simulink model "summary"  (R2022b)
settings: Solver=FixedStepAuto  StartTime=0.0  StopTime=100  FixedStep=0.1  RelTol=1e-3
values from neighbouring files (symbols this model uses):
  C_M = 1.1366    [init.m]
  C_T = 3.5611    [init.m]
  D_p = 0.1    [init.m]
  ModelInit_Att_qw = 0    [init.m]
  ModelInit_Att_qx = 1    [init.m]
  ModelInit_Att_qy = 0    [init.m]
  ModelInit_Att_qz = 0    [init.m]
  ModelInit_Pos_x = 0    [init.m]
  ModelInit_Pos_y = 0    [init.m]
  ModelInit_Pos_z = 0    [init.m]
  ModelParam_c_M = 1.779e-07*2    (= 3.558e-07)    [init.m]
  ModelParam_c_T = 1.105e-05    [init.m]
  ModelParam_d = 0.225    [init.m]
  ModelParam_g = 9.8    [init.m]
  ModelParam_I_xx = 0.0211    [init.m]
  ModelParam_I_yy = 0.0219    [init.m]
  ModelParam_I_zz = 0.0366    [init.m]
  ModelParam_J_RP = 0.0001287    [init.m]
  ModelParam_m = 1.4    [init.m]
  p = pos(idx,:)    [draw_morecool.m]    (also in init.m = 1.225)
libraries: mpclib x3
settings Model: Creator=12854  LastModifiedBy=12854
settings OptimizationCC: BlockReduction=off  DefaultParameterBehavior=Inlined  BufferReuse=off

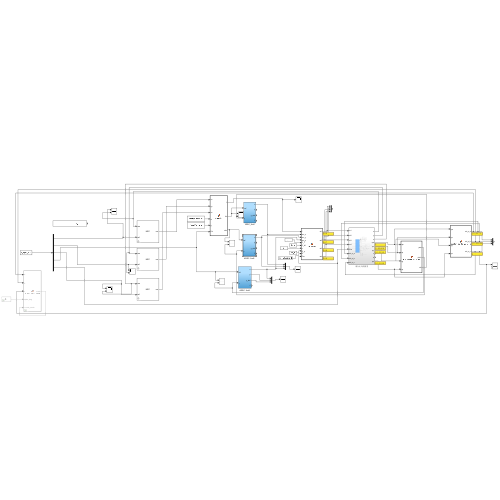
[thumbnail: Simulink's stored preview of the top-level diagram]
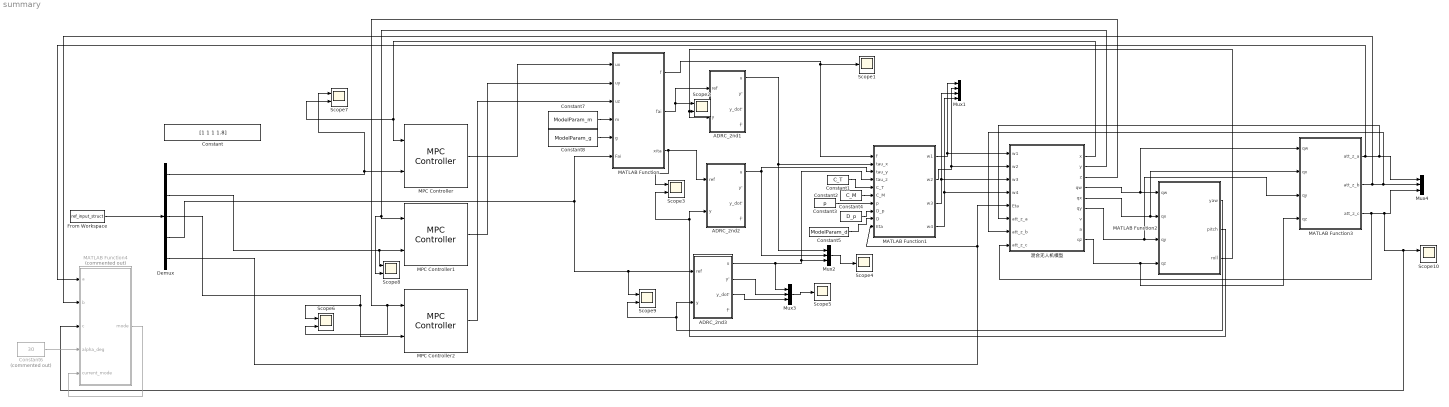
== system summary ==
  ADRC_2nd1 : Subsystem
  ADRC_2nd2 : Subsystem
  ADRC_2nd3 : Subsystem
  Constant : Constant  Value=[1 1 1 1.8]
  Constant1 : Constant  Value=C_T
  Constant2 : Constant  Value=C_M
  Constant3 : Constant  Value=p
  Constant4 : Constant  Value=D_p
  Constant5 : Constant  Value=ModelParam_d
  Constant6 : Constant  Commented=on  Value=30
  Constant7 : Constant  Value=ModelParam_m
  Constant8 : Constant  Value=ModelParam_g
  Demux : Demux  Outputs=5
  From Workspace : FromWorkspace  VariableName=ref_input_struct
  MATLAB Function : MATLAB Function  TreatAsAtomicUnit=on
  MATLAB Function1 : MATLAB Function  TreatAsAtomicUnit=on
  MATLAB Function2 : MATLAB Function  TreatAsAtomicUnit=on
  MATLAB Function3 : MATLAB Function  TreatAsAtomicUnit=on
  MATLAB Function4 : MATLAB Function  Commented=on  TreatAsAtomicUnit=on
  MPC Controller : mpclib/MPC Controller  SCDEnableBlockLinearizationSpecification=on  mpcobj=mpcobj_x  x0=[]  is_multiple=0  enable_value=0  return_u0=off  updateMPCinCallerWorkspace=on  md_inport=off  mv_inport=off  uref_inport=off  return_cost=off  return_mvseq=off  return_qpstatus=off  return_xseq=off  return_state=off  return_ovseq=off  state_inport=off  umin_inport=off  umax_inport=off  ymin_inport=off  ymax_inport=off  cc_inport=off  ywt_inport=off  uwt_inport=off  duwt_inport=off  rhoeps_inport=off  pm_inport=off  MaximumP=10  HorizonChoice=FixedHorizon  n_ts=0.1  n_p=10  n_mv=1  n_md=0  n_ud=0  n_mo=1  n_uo=0  BlockDataType=double  SampleTimeInherited=off  switch_inport=off
  MPC Controller1 : mpclib/MPC Controller  SCDEnableBlockLinearizationSpecification=on  mpcobj=mpcobj_y  x0=[]  is_multiple=0  enable_value=0  return_u0=off  updateMPCinCallerWorkspace=on  md_inport=off  mv_inport=off  uref_inport=off  return_cost=off  return_mvseq=off  return_qpstatus=off  return_xseq=off  return_state=off  return_ovseq=off  state_inport=off  umin_inport=off  umax_inport=off  ymin_inport=off  ymax_inport=off  cc_inport=off  ywt_inport=off  uwt_inport=off  duwt_inport=off  rhoeps_inport=off  pm_inport=off  MaximumP=10  HorizonChoice=FixedHorizon  n_ts=0.1  n_p=10  n_mv=1  n_md=0  n_ud=0  n_mo=1  n_uo=0  BlockDataType=double  SampleTimeInherited=off  switch_inport=off
  MPC Controller2 : mpclib/MPC Controller  SCDEnableBlockLinearizationSpecification=on  mpcobj=mpcobj_z  x0=[]  is_multiple=0  enable_value=0  return_u0=off  updateMPCinCallerWorkspace=on  md_inport=off  mv_inport=off  uref_inport=off  return_cost=off  return_mvseq=off  return_qpstatus=off  return_xseq=off  return_state=off  return_ovseq=off  state_inport=off  umin_inport=off  umax_inport=off  ymin_inport=off  ymax_inport=off  cc_inport=off  ywt_inport=off  uwt_inport=off  duwt_inport=off  rhoeps_inport=off  pm_inport=off  MaximumP=10  HorizonChoice=FixedHorizon  n_ts=0.1  n_p=10  n_mv=1  n_md=0  n_ud=0  n_mo=1  n_uo=0  BlockDataType=double  SampleTimeInherited=off  switch_inport=off
  Mux1 : Mux
  Mux2 : Mux  Inputs=3
  Mux3 : Mux  Inputs=3
  Mux4 : Mux  Inputs=3
  Scope1 : Scope
  Scope{2..3,6..10} (7 alike) : Scope  NumInputPorts=2
  Scope4 : Scope
  Scope5 : Scope
  混合无人机模型 : Subsystem
  wires:
  混合无人机模型/1(x) -> MPC Controller/1, Scope7/2
  混合无人机模型/2(y) -> Scope8/2, MPC Controller1/1
  混合无人机模型/3(z) -> Scope6/2, MPC Controller2/1
  Demux/1 -> Scope7/1, MPC Controller/2
  Demux/2 -> Scope8/1, MPC Controller1/2
  Demux/3 -> Scope6/1, MPC Controller2/2
  From Workspace/1 -> Demux/1
  MPC Controller/1 -> MATLAB Function/1(ux)
  MPC Controller1/1 -> MATLAB Function/2(uy)
  MPC Controller2/1 -> MATLAB Function/3(uz)
  Demux/4 -> MATLAB Function/6(Fai), Scope9/1, ADRC_2nd3/1(ref)
  Constant8/1 -> MATLAB Function/5(g)
  Constant7/1 -> MATLAB Function/4(m)
  MATLAB Function/1(f) -> Scope1/1, MATLAB Function1/1(f)
  MATLAB Function/2(fai) -> ADRC_2nd1/1(ref), Scope2/1
  MATLAB Function/3(xita) -> ADRC_2nd2/1(ref), Scope3/1
  ADRC_2nd3/1(u) -> Mux2/3, MATLAB Function1/4(tau_z), Mux3/1
  MATLAB Function1/1(w1) -> Mux1/1, 混合无人机模型/1(w1)
  MATLAB Function1/2(w2) -> 混合无人机模型/2(w2), Mux1/2
  MATLAB Function1/3(w3) -> 混合无人机模型/3(w3), Mux1/3
  MATLAB Function1/4(w4) -> 混合无人机模型/4(w4), Mux1/4
  Constant1/1 -> MATLAB Function1/5(C_T)
  Constant2/1 -> MATLAB Function1/6(C_M)
  Constant4/1 -> MATLAB Function1/8(D_p)
  Constant5/1 -> MATLAB Function1/9(D)
  Mux2/1 -> Scope4/1
  Mux3/1 -> Scope5/1
  ADRC_2nd3/2(y') -> Mux3/2
  ADRC_2nd3/3(y_dot') -> Mux3/3
  ADRC_2nd1/1(u) -> Mux2/1, MATLAB Function1/2(tau_x)
  ADRC_2nd2/1(u) -> Mux2/2, MATLAB Function1/3(tau_y)
  Constant3/1 -> MATLAB Function1/7(p)
  Demux/5 -> MATLAB Function1/10(Eta), 混合无人机模型/5(Eta)
  混合无人机模型/4(qw) -> MATLAB Function3/1(qw), MATLAB Function2/1(qw)
  混合无人机模型/5(qx) -> MATLAB Function3/2(qx), MATLAB Function2/2(qx)
  混合无人机模型/6(qy) -> MATLAB Function3/3(qy), MATLAB Function2/3(qy)
  混合无人机模型/9(qz) -> MATLAB Function3/4(qz), MATLAB Function2/4(qz)
  MATLAB Function2/3(roll) -> Scope2/2, ADRC_2nd1/2(y)
  MATLAB Function2/2(pitch) -> Scope3/2, ADRC_2nd2/2(y)
  MATLAB Function2/1(yaw) -> Scope9/2, ADRC_2nd3/2(y)
  MATLAB Function3/2(att_z_b) -> MATLAB Function4/2(b), 混合无人机模型/7(att_z_b), Mux4/2
  MATLAB Function3/3(att_z_c) -> 混合无人机模型/8(att_z_c), MATLAB Function4/3(c), Scope10/1, Mux4/3
  MATLAB Function4/1(mode) -> MATLAB Function4/5(current_mode)
  MATLAB Function3/1(att_z_a) -> MATLAB Function4/1(a), 混合无人机模型/6(att_z_a), Mux4/1
  Constant6/1 -> MATLAB Function4/4(alpha_deg)

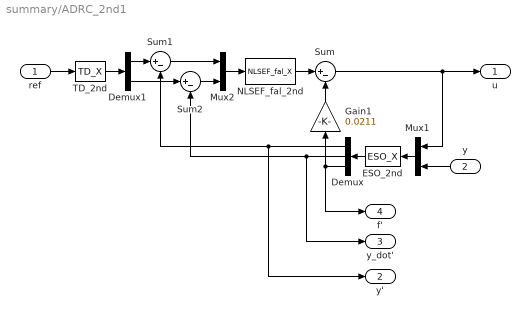
== system summary/ADRC_2nd1 ==
  ref : Inport
  y : Inport  Port=2
  Demux : Demux  Outputs=3
  Demux1 : Demux  Outputs=2
  ESO_2nd : S-Function  FunctionName=ESO_X  Parameters=CtrlParaX  SFunctionDeploymentMode=off  EnableBusSupport=off
  Gain1 : Gain  Gain=0.0211
  Mux1 : Mux  Inputs=2
  Mux2 : Mux  Inputs=2
  NLSEF_fal_2nd : S-Function  FunctionName=NLSEF_fal_X  Parameters=CtrlParaX  SFunctionDeploymentMode=off  EnableBusSupport=off
  Sum : Sum  Inputs=|+-
  Sum1 : Sum  Inputs=|+-
  Sum2 : Sum  Inputs=|+-
  TD_2nd : S-Function  FunctionName=TD_X  Parameters=CtrlParaX  SFunctionDeploymentMode=off  EnableBusSupport=off
  u : Outport  VectorParamsAs1DForOutWhenUnconnected=off
  y' : Outport  Port=2  VectorParamsAs1DForOutWhenUnconnected=off
  y_dot' : Outport  Port=3  VectorParamsAs1DForOutWhenUnconnected=off
  f' : Outport  Port=4  VectorParamsAs1DForOutWhenUnconnected=off
  wires:
  Mux2/1 -> NLSEF_fal_2nd/1
  ESO_2nd/1 -> Demux/1
  Demux1/2 -> Sum2/1
  ref/1 -> TD_2nd/1
  Demux/1 -> y'/1, Sum1/2
  TD_2nd/1 -> Demux1/1
  y/1 -> Mux1/2
  Gain1/1 -> Sum/2
  Demux/2 -> y_dot'/1, Sum2/2
  Demux1/1 -> Sum1/1
  Demux/3 -> Gain1/1, f'/1
  Sum2/1 -> Mux2/2
  Sum/1 -> Mux1/1, u/1
  NLSEF_fal_2nd/1 -> Sum/1
  Sum1/1 -> Mux2/1
  Mux1/1 -> ESO_2nd/1

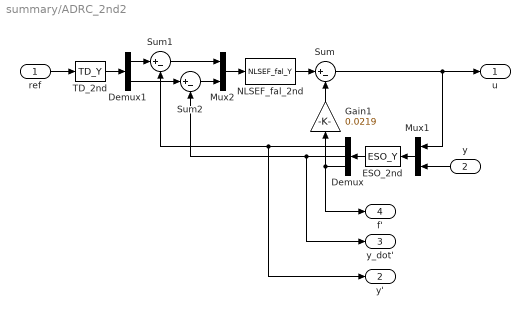
== system summary/ADRC_2nd2 ==
  ref : Inport
  y : Inport  Port=2
  Demux : Demux  Outputs=3
  Demux1 : Demux  Outputs=2
  ESO_2nd : S-Function  FunctionName=ESO_Y  Parameters=CtrlParaY  SFunctionDeploymentMode=off  EnableBusSupport=off
  Gain1 : Gain  Gain=0.0219
  Mux1 : Mux  Inputs=2
  Mux2 : Mux  Inputs=2
  NLSEF_fal_2nd : S-Function  FunctionName=NLSEF_fal_Y  Parameters=CtrlParaY  SFunctionDeploymentMode=off  EnableBusSupport=off
  Sum : Sum  Inputs=|+-
  Sum1 : Sum  Inputs=|+-
  Sum2 : Sum  Inputs=|+-
  TD_2nd : S-Function  FunctionName=TD_Y  Parameters=CtrlParaY  SFunctionDeploymentMode=off  EnableBusSupport=off
  u : Outport  VectorParamsAs1DForOutWhenUnconnected=off
  y' : Outport  Port=2  VectorParamsAs1DForOutWhenUnconnected=off
  y_dot' : Outport  Port=3  VectorParamsAs1DForOutWhenUnconnected=off
  f' : Outport  Port=4  VectorParamsAs1DForOutWhenUnconnected=off
  wires:
  Mux2/1 -> NLSEF_fal_2nd/1
  ESO_2nd/1 -> Demux/1
  Demux1/2 -> Sum2/1
  ref/1 -> TD_2nd/1
  Demux/1 -> y'/1, Sum1/2
  TD_2nd/1 -> Demux1/1
  y/1 -> Mux1/2
  Gain1/1 -> Sum/2
  Demux/2 -> y_dot'/1, Sum2/2
  Demux1/1 -> Sum1/1
  Demux/3 -> Gain1/1, f'/1
  Sum2/1 -> Mux2/2
  Sum/1 -> Mux1/1, u/1
  NLSEF_fal_2nd/1 -> Sum/1
  Sum1/1 -> Mux2/1
  Mux1/1 -> ESO_2nd/1

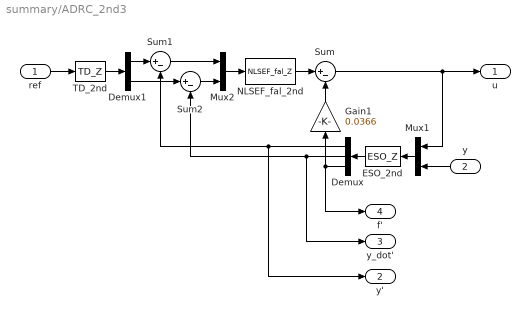
== system summary/ADRC_2nd3 ==
  ref : Inport
  y : Inport  Port=2
  Demux : Demux  Outputs=3
  Demux1 : Demux  Outputs=2
  ESO_2nd : S-Function  FunctionName=ESO_Z  Parameters=CtrlParaZ  SFunctionDeploymentMode=off  EnableBusSupport=off
  Gain1 : Gain  Gain=0.0366
  Mux1 : Mux  Inputs=2
  Mux2 : Mux  Inputs=2
  NLSEF_fal_2nd : S-Function  FunctionName=NLSEF_fal_Z  Parameters=CtrlParaZ  SFunctionDeploymentMode=off  EnableBusSupport=off
  Sum : Sum  Inputs=|+-
  Sum1 : Sum  Inputs=|+-
  Sum2 : Sum  Inputs=|+-
  TD_2nd : S-Function  FunctionName=TD_Z  Parameters=CtrlParaZ  SFunctionDeploymentMode=off  EnableBusSupport=off
  u : Outport  VectorParamsAs1DForOutWhenUnconnected=off
  y' : Outport  Port=2  VectorParamsAs1DForOutWhenUnconnected=off
  y_dot' : Outport  Port=3  VectorParamsAs1DForOutWhenUnconnected=off
  f' : Outport  Port=4  VectorParamsAs1DForOutWhenUnconnected=off
  wires:
  Mux2/1 -> NLSEF_fal_2nd/1
  ESO_2nd/1 -> Demux/1
  Demux1/2 -> Sum2/1
  ref/1 -> TD_2nd/1
  Demux/1 -> y'/1, Sum1/2
  TD_2nd/1 -> Demux1/1
  y/1 -> Mux1/2
  Gain1/1 -> Sum/2
  Demux/2 -> y_dot'/1, Sum2/2
  Demux1/1 -> Sum1/1
  Demux/3 -> Gain1/1, f'/1
  Sum2/1 -> Mux2/2
  Sum/1 -> Mux1/1, u/1
  NLSEF_fal_2nd/1 -> Sum/1
  Sum1/1 -> Mux2/1
  Mux1/1 -> ESO_2nd/1

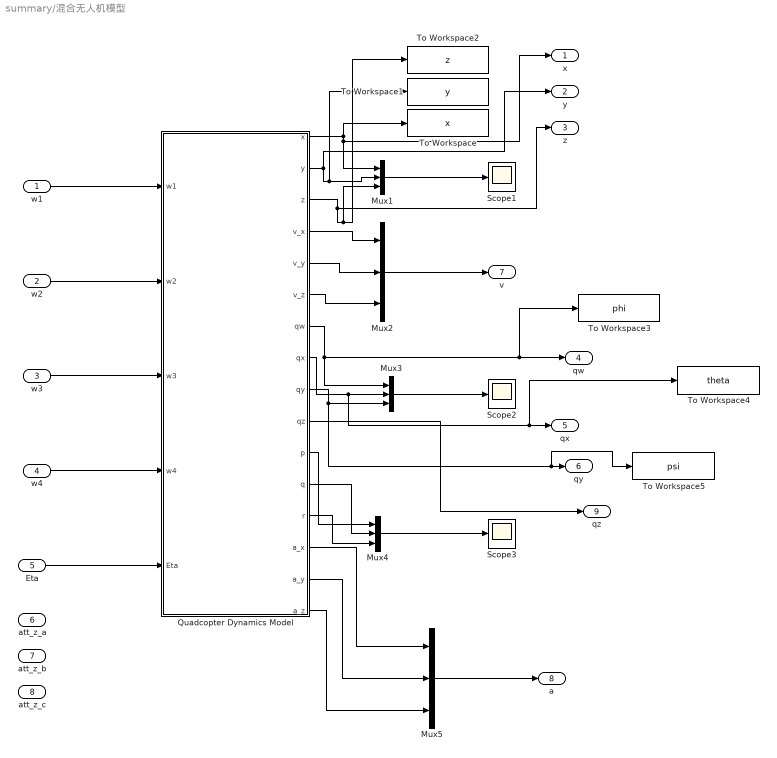
== system summary/混合无人机模型 ==
  w1 : Inport
  w2 : Inport  Port=2
  w3 : Inport  Port=3
  w4 : Inport  Port=4
  Eta : Inport  Port=5
  att_z_a : Inport  Port=6
  att_z_b : Inport  Port=7
  att_z_c : Inport  Port=8
  Mux{1..5} (5 alike) : Mux  Inputs=3
  Quadcopter Dynamics Model : Subsystem
  Scope1 : Scope
  Scope2 : Scope
  Scope3 : Scope
  To Workspace : ToWorkspace  VariableName=x  SaveFormat=Timeseries  SampleTime=-1
  To Workspace1 : ToWorkspace  VariableName=y  SaveFormat=Timeseries  SampleTime=-1
  To Workspace2 : ToWorkspace  VariableName=z  SaveFormat=Timeseries  SampleTime=-1
  To Workspace3 : ToWorkspace  VariableName=phi  SaveFormat=Timeseries  SampleTime=-1
  To Workspace4 : ToWorkspace  VariableName=theta  SaveFormat=Timeseries  SampleTime=-1
  To Workspace5 : ToWorkspace  VariableName=psi  SaveFormat=Timeseries  SampleTime=-1
  x : Outport
  y : Outport  Port=2
  z : Outport  Port=3
  qw : Outport  Port=4
  qx : Outport  Port=5
  qy : Outport  Port=6
  v : Outport  Port=7
  a : Outport  Port=8
  qz : Outport  Port=9
  wires:
  Mux4/1 -> Scope3/1
  Mux3/1 -> Scope2/1
  Quadcopter Dynamics Model/2(y) -> To Workspace1/1, Mux1/2, y/1
  Quadcopter Dynamics Model/8(qx) -> To Workspace4/1, qx/1, Mux3/2
  Quadcopter Dynamics Model/5(v_y) -> Mux2/2
  Quadcopter Dynamics Model/1(x) -> Mux1/1, x/1, To Workspace/1
  Quadcopter Dynamics Model/6(v_z) -> Mux2/3
  Mux2/1 -> v/1
  Quadcopter Dynamics Model/13(r) -> Mux4/3
  Mux1/1 -> Scope1/1
  Quadcopter Dynamics Model/11(p) -> Mux4/1
  Quadcopter Dynamics Model/4(v_x) -> Mux2/1
  Quadcopter Dynamics Model/7(qw) -> Mux3/1, To Workspace3/1, qw/1
  Quadcopter Dynamics Model/3(z) -> To Workspace2/1, Mux1/3, z/1
  Quadcopter Dynamics Model/12(q) -> Mux4/2
  Quadcopter Dynamics Model/9(qy) -> To Workspace5/1, qy/1, Mux3/3
  w1/1 -> Quadcopter Dynamics Model/1(w1)
  w2/1 -> Quadcopter Dynamics Model/2(w2)
  w3/1 -> Quadcopter Dynamics Model/3(w3)
  w4/1 -> Quadcopter Dynamics Model/4(w4)
  Quadcopter Dynamics Model/16(a_z) -> Mux5/3
  Quadcopter Dynamics Model/15(a_y) -> Mux5/2
  Quadcopter Dynamics Model/14(a_x) -> Mux5/1
  Mux5/1 -> a/1
  Quadcopter Dynamics Model/10(qz) -> qz/1
  Eta/1 -> Quadcopter Dynamics Model/5(Eta)

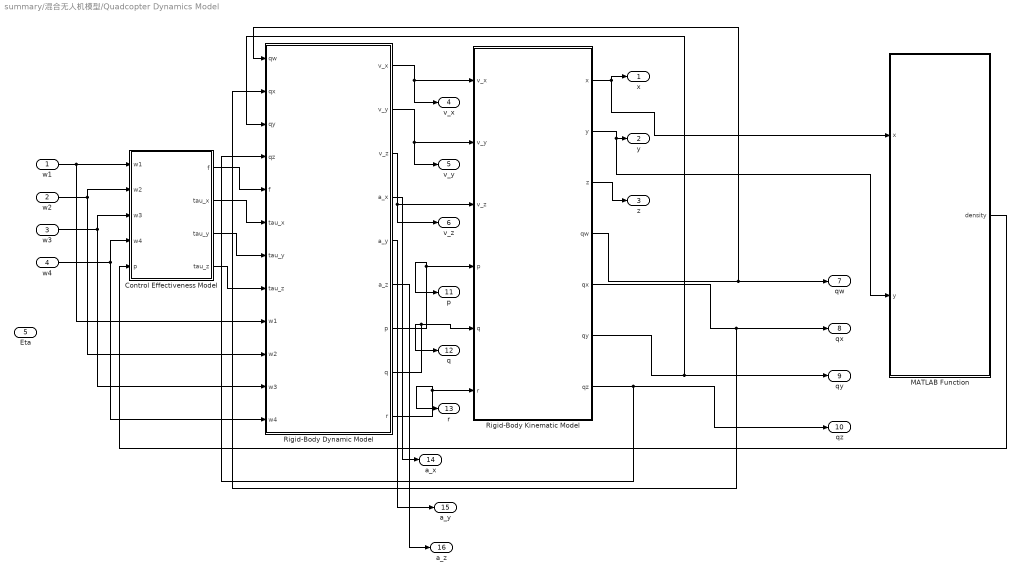
== system summary/混合无人机模型/Quadcopter Dynamics Model ==
  w1 : Inport
  w2 : Inport  Port=2
  w3 : Inport  Port=3
  w4 : Inport  Port=4
  Eta : Inport  Port=5
  Control Effectiveness Model : Subsystem
  MATLAB Function : MATLAB Function  TreatAsAtomicUnit=on
  Rigid-Body Dynamic Model : Subsystem
  Rigid-Body Kinematic Model : Subsystem
  x : Outport  VectorParamsAs1DForOutWhenUnconnected=off
  y : Outport  Port=2  VectorParamsAs1DForOutWhenUnconnected=off
  z : Outport  Port=3  VectorParamsAs1DForOutWhenUnconnected=off
  v_x : Outport  Port=4  VectorParamsAs1DForOutWhenUnconnected=off
  v_y : Outport  Port=5  VectorParamsAs1DForOutWhenUnconnected=off
  v_z : Outport  Port=6  VectorParamsAs1DForOutWhenUnconnected=off
  qw : Outport  Port=7  VectorParamsAs1DForOutWhenUnconnected=off
  qx : Outport  Port=8  VectorParamsAs1DForOutWhenUnconnected=off
  qy : Outport  Port=9  VectorParamsAs1DForOutWhenUnconnected=off
  qz : Outport  Port=10  VectorParamsAs1DForOutWhenUnconnected=off
  p : Outport  Port=11  VectorParamsAs1DForOutWhenUnconnected=off
  q : Outport  Port=12  VectorParamsAs1DForOutWhenUnconnected=off
  r : Outport  Port=13  VectorParamsAs1DForOutWhenUnconnected=off
  a_x : Outport  Port=14  VectorParamsAs1DForOutWhenUnconnected=off
  a_y : Outport  Port=15  VectorParamsAs1DForOutWhenUnconnected=off
  a_z : Outport  Port=16  VectorParamsAs1DForOutWhenUnconnected=off
  wires:
  w1/1 -> Rigid-Body Dynamic Model/9(w1), Control Effectiveness Model/1(w1)
  w3/1 -> Rigid-Body Dynamic Model/11(w3), Control Effectiveness Model/3(w3)
  w4/1 -> Rigid-Body Dynamic Model/12(w4), Control Effectiveness Model/4(w4)
  w2/1 -> Control Effectiveness Model/2(w2), Rigid-Body Dynamic Model/10(w2)
  Rigid-Body Dynamic Model/7(p) -> p/1, Rigid-Body Kinematic Model/4(p)
  Rigid-Body Dynamic Model/9(r) -> r/1, Rigid-Body Kinematic Model/6(r)
  Control Effectiveness Model/2(tau_x) -> Rigid-Body Dynamic Model/6(tau_x)
  Rigid-Body Kinematic Model/1(x) -> x/1, MATLAB Function/1(x)
  Rigid-Body Dynamic Model/8(q) -> q/1, Rigid-Body Kinematic Model/5(q)
  Control Effectiveness Model/4(tau_z) -> Rigid-Body Dynamic Model/8(tau_z)
  Rigid-Body Kinematic Model/2(y) -> MATLAB Function/2(y), y/1
  Rigid-Body Kinematic Model/3(z) -> z/1
  Control Effectiveness Model/3(tau_y) -> Rigid-Body Dynamic Model/7(tau_y)
  Rigid-Body Kinematic Model/4(qw) -> Rigid-Body Dynamic Model/1(qw), qw/1
  Rigid-Body Kinematic Model/5(qx) -> Rigid-Body Dynamic Model/2(qx), qx/1
  Rigid-Body Kinematic Model/6(qy) -> Rigid-Body Dynamic Model/3(qy), qy/1
  MATLAB Function/1(density) -> Control Effectiveness Model/5(p)
  Rigid-Body Dynamic Model/4(a_x) -> a_x/1
  Rigid-Body Dynamic Model/5(a_y) -> a_y/1
  Rigid-Body Dynamic Model/6(a_z) -> a_z/1
  Rigid-Body Dynamic Model/1(v_x) -> Rigid-Body Kinematic Model/1(v_x), v_x/1
  Rigid-Body Dynamic Model/2(v_y) -> Rigid-Body Kinematic Model/2(v_y), v_y/1
  Rigid-Body Dynamic Model/3(v_z) -> Rigid-Body Kinematic Model/3(v_z), v_z/1
  Control Effectiveness Model/1(f) -> Rigid-Body Dynamic Model/5(f)
  Rigid-Body Kinematic Model/7(qz) -> Rigid-Body Dynamic Model/4(qz), qz/1

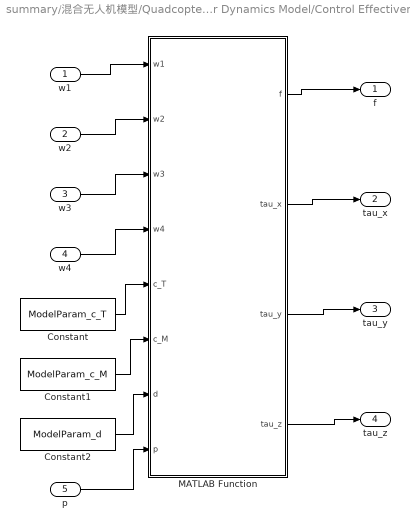
== system summary/混合无人机模型/Quadcopter Dynamics Model/Control Effectiveness Model ==
  w1 : Inport
  w2 : Inport  Port=2
  w3 : Inport  Port=3
  w4 : Inport  Port=4
  p : Inport  Port=5
  Constant : Constant  Value=ModelParam_c_T
  Constant1 : Constant  Value=ModelParam_c_M
  Constant2 : Constant  Value=ModelParam_d
  MATLAB Function : MATLAB Function  TreatAsAtomicUnit=on
  f : Outport  VectorParamsAs1DForOutWhenUnconnected=off
  tau_x : Outport  Port=2  VectorParamsAs1DForOutWhenUnconnected=off
  tau_y : Outport  Port=3  VectorParamsAs1DForOutWhenUnconnected=off
  tau_z : Outport  Port=4  VectorParamsAs1DForOutWhenUnconnected=off
  wires:
  Constant1/1 -> MATLAB Function/6(c_M)
  Constant/1 -> MATLAB Function/5(c_T)
  MATLAB Function/3(tau_y) -> tau_y/1
  MATLAB Function/1(f) -> f/1
  Constant2/1 -> MATLAB Function/7(d)
  MATLAB Function/4(tau_z) -> tau_z/1
  w3/1 -> MATLAB Function/3(w3)
  w1/1 -> MATLAB Function/1(w1)
  w4/1 -> MATLAB Function/4(w4)
  MATLAB Function/2(tau_x) -> tau_x/1
  w2/1 -> MATLAB Function/2(w2)
  p/1 -> MATLAB Function/8(p)

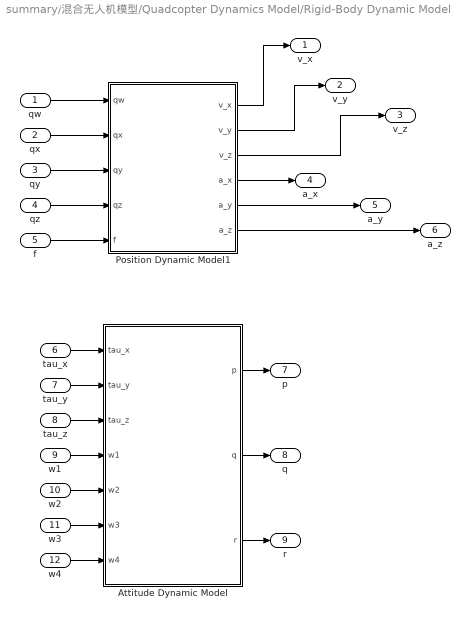
== system summary/混合无人机模型/Quadcopter Dynamics Model/Rigid-Body Dynamic Model ==
  qw : Inport
  qx : Inport  Port=2
  qy : Inport  Port=3
  qz : Inport  Port=4
  f : Inport  Port=5
  tau_x : Inport  Port=6
  tau_y : Inport  Port=7
  tau_z : Inport  Port=8
  w1 : Inport  Port=9
  w2 : Inport  Port=10
  w3 : Inport  Port=11
  w4 : Inport  Port=12
  Attitude Dynamic Model : Subsystem
  Position Dynamic Model1 : Subsystem
  v_x : Outport  VectorParamsAs1DForOutWhenUnconnected=off
  v_y : Outport  Port=2  VectorParamsAs1DForOutWhenUnconnected=off
  v_z : Outport  Port=3  VectorParamsAs1DForOutWhenUnconnected=off
  a_x : Outport  Port=4  VectorParamsAs1DForOutWhenUnconnected=off
  a_y : Outport  Port=5  VectorParamsAs1DForOutWhenUnconnected=off
  a_z : Outport  Port=6  VectorParamsAs1DForOutWhenUnconnected=off
  p : Outport  Port=7  VectorParamsAs1DForOutWhenUnconnected=off
  q : Outport  Port=8  VectorParamsAs1DForOutWhenUnconnected=off
  r : Outport  Port=9  VectorParamsAs1DForOutWhenUnconnected=off
  wires:
  w3/1 -> Attitude Dynamic Model/6(w3)
  w1/1 -> Attitude Dynamic Model/4(w1)
  tau_x/1 -> Attitude Dynamic Model/1(tau_x)
  w2/1 -> Attitude Dynamic Model/5(w2)
  Attitude Dynamic Model/1(p) -> p/1
  w4/1 -> Attitude Dynamic Model/7(w4)
  Attitude Dynamic Model/2(q) -> q/1
  tau_y/1 -> Attitude Dynamic Model/2(tau_y)
  tau_z/1 -> Attitude Dynamic Model/3(tau_z)
  Attitude Dynamic Model/3(r) -> r/1
  qw/1 -> Position Dynamic Model1/1(qw)
  qx/1 -> Position Dynamic Model1/2(qx)
  qy/1 -> Position Dynamic Model1/3(qy)
  qz/1 -> Position Dynamic Model1/4(qz)
  f/1 -> Position Dynamic Model1/5(f)
  Position Dynamic Model1/1(v_x) -> v_x/1
  Position Dynamic Model1/2(v_y) -> v_y/1
  Position Dynamic Model1/3(v_z) -> v_z/1
  Position Dynamic Model1/4(a_x) -> a_x/1
  Position Dynamic Model1/5(a_y) -> a_y/1
  Position Dynamic Model1/6(a_z) -> a_z/1

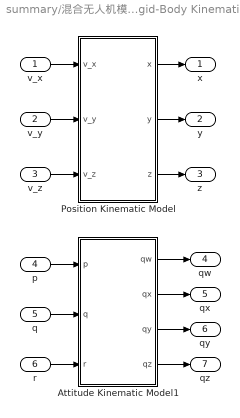
== system summary/混合无人机模型/Quadcopter Dynamics Model/Rigid-Body Kinematic Model ==
  v_x : Inport
  v_y : Inport  Port=2
  v_z : Inport  Port=3
  p : Inport  Port=4
  q : Inport  Port=5
  r : Inport  Port=6
  Attitude Kinematic Model1 : Subsystem
  Position Kinematic Model : Subsystem
  x : Outport  VectorParamsAs1DForOutWhenUnconnected=off
  y : Outport  Port=2  VectorParamsAs1DForOutWhenUnconnected=off
  z : Outport  Port=3  VectorParamsAs1DForOutWhenUnconnected=off
  qw : Outport  Port=4  VectorParamsAs1DForOutWhenUnconnected=off
  qx : Outport  Port=5  VectorParamsAs1DForOutWhenUnconnected=off
  qy : Outport  Port=6  VectorParamsAs1DForOutWhenUnconnected=off
  qz : Outport  Port=7  VectorParamsAs1DForOutWhenUnconnected=off
  wires:
  v_x/1 -> Position Kinematic Model/1(v_x)
  v_y/1 -> Position Kinematic Model/2(v_y)
  r/1 -> Attitude Kinematic Model1/3(r)
  p/1 -> Attitude Kinematic Model1/1(p)
  v_z/1 -> Position Kinematic Model/3(v_z)
  Position Kinematic Model/1(x) -> x/1
  Position Kinematic Model/2(y) -> y/1
  q/1 -> Attitude Kinematic Model1/2(q)
  Position Kinematic Model/3(z) -> z/1
  Attitude Kinematic Model1/2(qx) -> qx/1
  Attitude Kinematic Model1/1(qw) -> qw/1
  Attitude Kinematic Model1/3(qy) -> qy/1
  Attitude Kinematic Model1/4(qz) -> qz/1

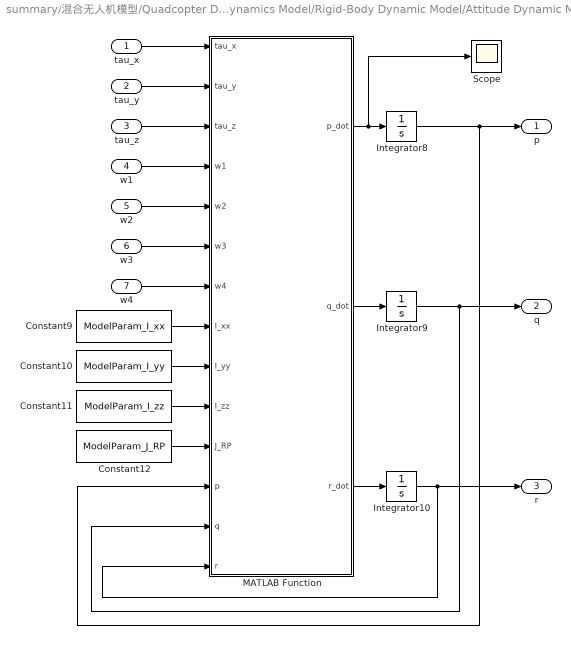
== system summary/混合无人机模型/Quadcopter Dynamics Model/Rigid-Body Dynamic Model/Attitude Dynamic Model ==
  tau_x : Inport
  tau_y : Inport  Port=2
  tau_z : Inport  Port=3
  w1 : Inport  Port=4
  w2 : Inport  Port=5
  w3 : Inport  Port=6
  w4 : Inport  Port=7
  Constant10 : Constant  Value=ModelParam_I_yy
  Constant11 : Constant  Value=ModelParam_I_zz
  Constant12 : Constant  Value=ModelParam_J_RP
  Constant9 : Constant  Value=ModelParam_I_xx
  Integrator10 : Integrator
  Integrator8 : Integrator
  Integrator9 : Integrator
  MATLAB Function : MATLAB Function  TreatAsAtomicUnit=on
  Scope : Scope
  p : Outport  VectorParamsAs1DForOutWhenUnconnected=off
  q : Outport  Port=2  VectorParamsAs1DForOutWhenUnconnected=off
  r : Outport  Port=3  VectorParamsAs1DForOutWhenUnconnected=off
  wires:
  Constant9/1 -> MATLAB Function/8(I_xx)
  tau_z/1 -> MATLAB Function/3(tau_z)
  Integrator10/1 -> r/1, MATLAB Function/14(r)
  Constant12/1 -> MATLAB Function/11(J_RP)
  Integrator9/1 -> q/1, MATLAB Function/13(q)
  Constant10/1 -> MATLAB Function/9(I_yy)
  MATLAB Function/3(r_dot) -> Integrator10/1
  MATLAB Function/1(p_dot) -> Scope/1, Integrator8/1
  Integrator8/1 -> p/1, MATLAB Function/12(p)
  tau_y/1 -> MATLAB Function/2(tau_y)
  MATLAB Function/2(q_dot) -> Integrator9/1
  Constant11/1 -> MATLAB Function/10(I_zz)
  w1/1 -> MATLAB Function/4(w1)
  tau_x/1 -> MATLAB Function/1(tau_x)
  w2/1 -> MATLAB Function/5(w2)
  w3/1 -> MATLAB Function/6(w3)
  w4/1 -> MATLAB Function/7(w4)

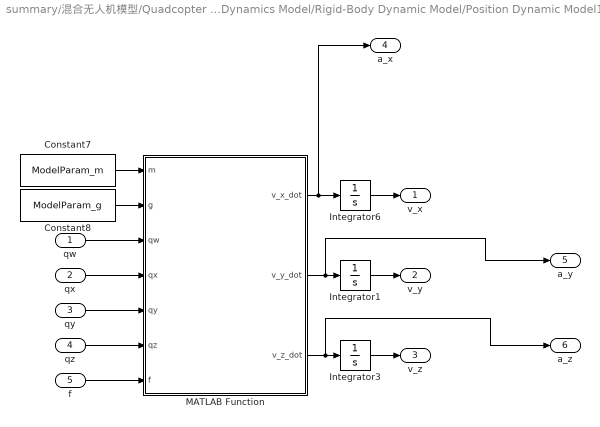
== system summary/混合无人机模型/Quadcopter Dynamics Model/Rigid-Body Dynamic Model/Position Dynamic Model1 ==
  qw : Inport
  qx : Inport  Port=2
  qy : Inport  Port=3
  qz : Inport  Port=4
  f : Inport  Port=5
  Constant7 : Constant  Value=ModelParam_m
  Constant8 : Constant  Value=ModelParam_g
  Integrator1 : Integrator
  Integrator3 : Integrator
  Integrator6 : Integrator
  MATLAB Function : MATLAB Function  TreatAsAtomicUnit=on
  v_x : Outport  VectorParamsAs1DForOutWhenUnconnected=off
  v_y : Outport  Port=2  VectorParamsAs1DForOutWhenUnconnected=off
  v_z : Outport  Port=3  VectorParamsAs1DForOutWhenUnconnected=off
  a_x : Outport  Port=4  VectorParamsAs1DForOutWhenUnconnected=off
  a_y : Outport  Port=5  VectorParamsAs1DForOutWhenUnconnected=off
  a_z : Outport  Port=6  VectorParamsAs1DForOutWhenUnconnected=off
  wires:
  Constant8/1 -> MATLAB Function/2(g)
  MATLAB Function/1(v_x_dot) -> a_x/1, Integrator6/1
  MATLAB Function/2(v_y_dot) -> a_y/1, Integrator1/1
  qx/1 -> MATLAB Function/4(qx)
  Constant7/1 -> MATLAB Function/1(m)
  MATLAB Function/3(v_z_dot) -> a_z/1, Integrator3/1
  qw/1 -> MATLAB Function/3(qw)
  f/1 -> MATLAB Function/7(f)
  qy/1 -> MATLAB Function/5(qy)
  Integrator6/1 -> v_x/1
  Integrator1/1 -> v_y/1
  Integrator3/1 -> v_z/1
  qz/1 -> MATLAB Function/6(qz)

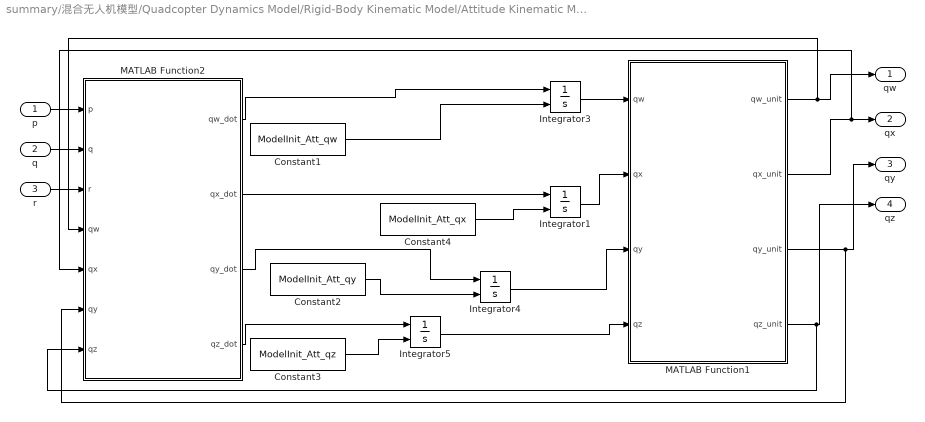
== system summary/混合无人机模型/Quadcopter Dynamics Model/Rigid-Body Kinematic Model/Attitude Kinematic Model1 ==
  p : Inport
  q : Inport  Port=2
  r : Inport  Port=3
  Constant1 : Constant  Value=ModelInit_Att_qw
  Constant2 : Constant  Value=ModelInit_Att_qy
  Constant3 : Constant  Value=ModelInit_Att_qz
  Constant4 : Constant  Value=ModelInit_Att_qx
  Integrator{1,3..5} (4 alike) : Integrator  InitialConditionSource=external
  MATLAB Function1 : MATLAB Function  TreatAsAtomicUnit=on
  MATLAB Function2 : MATLAB Function  TreatAsAtomicUnit=on
  qw : Outport  VectorParamsAs1DForOutWhenUnconnected=off
  qx : Outport  Port=2  VectorParamsAs1DForOutWhenUnconnected=off
  qy : Outport  Port=3  VectorParamsAs1DForOutWhenUnconnected=off
  qz : Outport  Port=4  VectorParamsAs1DForOutWhenUnconnected=off
  wires:
  r/1 -> MATLAB Function2/3(r)
  MATLAB Function2/1(qw_dot) -> Integrator3/1
  q/1 -> MATLAB Function2/2(q)
  p/1 -> MATLAB Function2/1(p)
  Constant1/1 -> Integrator3/2
  Constant2/1 -> Integrator4/2
  Constant3/1 -> Integrator5/2
  MATLAB Function2/2(qx_dot) -> Integrator1/1
  Constant4/1 -> Integrator1/2
  MATLAB Function2/3(qy_dot) -> Integrator4/1
  MATLAB Function2/4(qz_dot) -> Integrator5/1
  Integrator3/1 -> MATLAB Function1/1(qw)
  Integrator1/1 -> MATLAB Function1/2(qx)
  Integrator4/1 -> MATLAB Function1/3(qy)
  Integrator5/1 -> MATLAB Function1/4(qz)
  MATLAB Function1/1(qw_unit) -> MATLAB Function2/4(qw), qw/1
  MATLAB Function1/2(qx_unit) -> MATLAB Function2/5(qx), qx/1
  MATLAB Function1/3(qy_unit) -> MATLAB Function2/6(qy), qy/1
  MATLAB Function1/4(qz_unit) -> MATLAB Function2/7(qz), qz/1

== system summary/混合无人机模型/Quadcopter Dynamics Model/Rigid-Body Kinematic Model/Position Kinematic Model ==
  v_x : Inport
  v_y : Inport  Port=2
  v_z : Inport  Port=3
  Constant1 : Constant  Value=ModelInit_Pos_z
  Constant2 : Constant  Value=ModelInit_Pos_y
  Constant3 : Constant  Value=ModelInit_Pos_x
  Integrator : Integrator  InitialConditionSource=external
  Integrator1 : Integrator  InitialConditionSource=external
  Integrator2 : Integrator  InitialConditionSource=external
  x : Outport  VectorParamsAs1DForOutWhenUnconnected=off
  y : Outport  Port=2  VectorParamsAs1DForOutWhenUnconnected=off
  z : Outport  Port=3  VectorParamsAs1DForOutWhenUnconnected=off
  wires:
  v_z/1 -> Integrator2/1
  Integrator1/1 -> y/1
  Integrator/1 -> x/1
  Constant1/1 -> Integrator2/2
  Integrator2/1 -> z/1
  v_x/1 -> Integrator/1
  v_y/1 -> Integrator1/1
  Constant2/1 -> Integrator1/2
  Constant3/1 -> Integrator/2

== matlab function summary/混合无人机模型/Quadcopter Dynamics Model/Control Effectiveness Model/MATLAB Function ==
  data: w1 input; f output; w2 input; w3 input; w4 input; c_T input; c_M input; d input; tau_x output; tau_y output; tau_z output; p input
function [f, tau_x, tau_y, tau_z] = fcn(w1, w2, w3, w4, c_T, c_M, d, p)
% 函数描述
% 1.作用：本函数用来计算螺旋桨旋转产生的总拉力和反扭力矩。
% 2.函数输入：
%   wi：四个螺旋桨的转速(rad/s)，可以为正或负
%   c_T：螺旋桨拉力系数
%   c_M：螺旋桨转矩系数
%   d：机体中心和任一电机的距离(m)
% 3.函数输出：
%   f：螺旋桨拉力（机体轴）
%   tau_x：x轴反扭力矩（机体轴）
%   tau_y：y轴反扭力矩（机体轴）
%   tau_z：z轴反扭力矩（机体轴）
% 4.四旋翼构型为“X”型

% 计算每个螺旋桨产生的推力影响，考虑转速正负
f = p*c_T * (sign(w1)*w1^2 + sign(w2)*w2^2 + sign(w3)*w3^2 + sign(w4)*w4^2);
% 计算x轴扭矩，考虑螺旋桨的位置和旋转方向
tau_x = p*d * c_T * (sqrt(2)/2) * (sign(w1)*w1^2 - sign(w2)*w2^2 - sign(w3)*w3^2 + sign(w4)*w4^2);
% 计算y轴扭矩
tau_y = p*d * c_T * (sqrt(2)/2) * (sign(w1)*w1^2 + sign(w2)*w2^2 - sign(w3)*w3^2 - sign(w4)*w4^2);
% 计算z轴扭矩，只考虑螺旋桨转速和旋转方向
tau_z = p*c_M * (sign(w1)*w1^2 - sign(w2)*w2^2 + sign(w3)*w3^2 - sign(w4)*w4^2);

end

== matlab function summary/混合无人机模型/Quadcopter Dynamics Model/MATLAB Function ==
  data: x input; density output; y input
function density = air_density(x, y)
    % 定义火坑的中心位置
    center_x = 10;
    center_y = 10;

    % 定义火坑的半径
    radius = 3;

    % 定义火坑中心的空气密度为1.078 kg/m³
    density_center = 1.078;

    % 定义火坑边缘的空气密度为日常密度值
    density_edge = 1.225;

    % 计算无人机到火坑中心的距离
    r = sqrt((x - center_x)^2 + (y - center_y)^2);

    % 定义高斯函数的标准差
    sigma = radius / 3;
    
    % 使用高斯函数计算空气密度
    density = density_edge + (density_center - density_edge) * exp(-(r.^2) / (2 * sigma^2));


    density = density/1.225;
end

== matlab function summary/混合无人机模型/Quadcopter Dynamics Model/Rigid-Body Dynamic Model/Attitude Dynamic Model/MATLAB Function ==
  data: tau_x input; p_dot output; tau_y input; tau_z input; w1 input; w2 input; w3 input; w4 input; I_xx input; I_yy input; I_zz input; J_RP input; p input; q input; r input; q_dot output; r_dot output
function [p_dot, q_dot, r_dot] = fcn(tau_x, tau_y, tau_z, w1, w2, w3, w4, I_xx, I_yy, I_zz, J_RP, p, q, r)
% 函数描述
% 1.作用：本函数为四旋翼的姿态动力学微分方程组，通过四旋翼所受力矩和螺旋
%         桨转速计算得到四旋翼的机体角速度
% 2.函数输入：
%   wi：四个螺旋桨的转速(rad/s)
%   tau_x：x轴反扭力矩（机体轴）(N·m)
%   tau_y：y轴反扭力矩（机体轴）(N·m)
%   tau_z：z轴反扭力矩（机体轴）(N·m)
%   I_xx：四旋翼x轴转动惯量(kg·m^2)
%   I_yy：四旋翼y轴转动惯量(kg·m^2)
%   I_zz：四旋翼z轴转动惯量(kg·m^2)
%   J_RP：整个电机转子和螺旋桨绕转轴的总转动惯量(kg·m^2)
%   p：四旋翼x轴角速度（机体轴)(rad/s)
%   q：四旋翼y轴角速度（机体轴)(rad/s)
%   r：四旋翼z轴角速度（机体轴)(rad/s)
% 3.函数输出：
%   p_dot：四旋翼x轴角加速度（机体轴)
%   q_dot：四旋翼y轴角加速度（机体轴)
%   r_dot：四旋翼z轴角加速度（机体轴)
% 4.四旋翼构型为“X”型，螺旋桨序号如下所示：
%            1↑   2↓
%              \ /
%              / \
%            4↓   3↑
%   其中，↑表示螺旋桨逆时针旋转；↓表示螺旋桨顺时针旋转。

Omega = -w1 + w2 - w3 + w4;
p_dot = (1/I_xx) * (tau_x + q * r * (I_yy - I_zz) - J_RP * q * Omega);
q_dot = (1/I_yy) * (tau_y + p * r * (I_zz - I_xx) + J_RP * p * Omega);
r_dot = (1/I_zz) * (tau_z + p * q * (I_xx - I_yy) );
end

== matlab function summary/混合无人机模型/Quadcopter Dynamics Model/Rigid-Body Kinematic Model/Attitude Kinematic Model1/MATLAB Function2 ==
  data: p input; qw_dot output; q input; r input; qw input; qx input; qy input; qz input; qx_dot output; qy_dot output; qz_dot output
function [qw_dot, qx_dot, qy_dot, qz_dot] = updateQuaternion(p, q, r, qw, qx, qy, qz)
    % updateQuaternion 更新无人机的姿态四元数
    % 输入:
    %   q - 当前姿态四元数，形式为 [qw, qx, qy, qz]
    %   omega - 三轴角速度，形式为 [omega_x, omega_y, omega_z]
    %   dt - 时间步长

    % 将角速度转换为四元数形式
    q_current = [qw, qx, qy, qz];
    omega_q = [0, p, q, r];
    
    % 计算四元数的导数
    q_dot = 0.5 * quatmultiply(omega_q, q_current);
    qw_dot = q_dot(1);
    qx_dot = q_dot(2);
    qy_dot = q_dot(3);
    qz_dot = q_dot(4);
end

== matlab function summary/混合无人机模型/Quadcopter Dynamics Model/Rigid-Body Dynamic Model/Position Dynamic Model1/MATLAB Function ==
  data: m input; g input; qw input; qx input; qy input; qz input; f input; v_x_dot output; v_y_dot output; v_z_dot output
function [v_x_dot, v_y_dot, v_z_dot] = fcn(m, g, qw, qx, qy, qz, f)
% 函数描述
% 1.作用：本函数为四旋翼的位置动力学微分方程组，通过四旋翼所受拉力、姿态角
%         计算得到四旋翼飞行器的加速度
% 2.函数输入：
%   m：四旋翼飞行器质量(kg)
%   g：重力加速度(m/s^2)
%   qw：四元数1号位
%   qx：四元数2号位
%   qy：四元数3号位
%   qz：四元数4号位
%   f：螺旋桨产生的总拉力(N)
% 3.函数输出：
%   v_x_dot：地球坐标系下沿x轴的速度的导数
%   v_y_dot：地球坐标系下沿y轴的速度的导数
%   v_z_dot：地球坐标系下沿z轴的速度的导数
% 4.四旋翼构型为“X”型，螺旋桨序号如下所示：
%            3↓   1↑
%              \ /
%              / \
%            2↑   4↓
%   其中，↑表示螺旋桨逆时针旋转；↓表示螺旋桨顺时针旋转。
% 计算旋转矩阵 R
R11 = 1 - 2*qy^2 - 2*qz^2;
R12 = 2*qx*qy - 2*qz*qw;
R13 = 2*qx*qz + 2*qy*qw;
R21 = 2*qx*qy + 2*qz*qw;
R22 = 1 - 2*qx^2 - 2*qz^2;
R23 = 2*qy*qz - 2*qx*qw;
R31 = 2*qx*qz - 2*qy*qw;
R32 = 2*qy*qz + 2*qx*qw;
R33 = 1 - 2*qx^2 - 2*qy^2;

v_x_dot = -f * (1/m) * (R13);
v_y_dot = -f * (1/m) * (R23);
v_z_dot = g - f * (1/m) * R33;
end

== matlab function summary/MATLAB Function2 ==
  data: qw input; yaw output; qx input; qy input; pitch output; roll output; qz input
function [yaw, pitch, roll] = quaternion_to_euler(qw, qx, qy, qz)
    % 计算欧拉角
    % 偏航角
    yaw = atan2(2*(qw*qz + qx*qy), 1 - 2*(qy^2 + qz^2));
    % 俯仰角
    pitch = asin(2*(qw*qy - qz*qx));
    % 横滚角
    roll = atan2(2*(qw*qx + qy*qz), 1 - 2*(qx^2 + qy^2));

    % 将角度从弧度转换为度（如果需要）
    % yaw = rad2deg(yaw);
    % pitch = rad2deg(pitch);
    % roll = rad2deg(roll);
end

== matlab function summary/MATLAB Function3 ==
  data: qw input; att_z_a output; qx input; qy input; att_z_b output; att_z_c output; qz input
function [att_z_a, att_z_b, att_z_c] = quaternion_to_world_z(qw, qx, qy, qz)
    % 四元数表示的向量 (0, 0, 1)
    v = [0; 0; 1];
    
    % 四元数 q 和它的共轭 q*
    q = [qw, qx, qy, qz];
    q_conj = [qw, -qx, -qy, -qz];
    
    % 将向量 v 嵌入到四元数中，实部为 0
    v_q = [0, v'];
    
    % 执行四元数乘法 q * v_q * q*
    v_rotated = quatmultiply(q, quatmultiply(v_q, q_conj));
    
    % 输出变换后的向量组件
    att_z_a = v_rotated(2);
    att_z_b = v_rotated(3);
    att_z_c = v_rotated(4);
end

== matlab function summary/MATLAB Function ==
  data: ux input; f output; uy input; uz input; fai output; xita output; m input; g input; Fai input
function [f, fai, xita] = converter(ux, uy, uz, m, g, Fai)
%将加速度ux uy uz换算成推力和参考滚转角、俯仰角
%需要的参数有 无人机质量m、重力加速度g、参考偏航角Fai
f = m * sqrt((ux)^2+uy^2+(uz-g)^2);
fai = asin((-m)/f*((ux)*sin(Fai)-uy*cos(Fai)));
xita = atan(1/(uz-g)*((ux)*cos(Fai)+uy*sin(Fai)));

end

== matlab function summary/混合无人机模型/Quadcopter Dynamics Model/Rigid-Body Kinematic Model/Attitude Kinematic Model1/MATLAB Function1 ==
  data: qw_unit output; qw input; qx input; qy input; qz input; qx_unit output; qy_unit output; qz_unit output
function [qw_unit, qx_unit, qy_unit, qz_unit] = normalize_quaternion(qw, qx, qy, qz)
    % 计算四元数的模
    norm_q = sqrt(qw^2 + qx^2 + qy^2 + qz^2);
    
    % 检查模是否为零，避免除以零的错误
    if norm_q == 0
        error('Zero norm quaternion cannot be normalized.');
    end

    % 单位化四元数
    qw_unit = qw / norm_q;
    qx_unit = qx / norm_q;
    qy_unit = qy / norm_q;
    qz_unit = qz / norm_q;
end

== matlab function summary/MATLAB Function4 ==
  data: a input; mode output; b input; c input; alpha_deg input; current_mode input
function mode = checkModeSwitch(a, b, c, alpha_deg, current_mode)
    % a, b, c 是无人机机体z轴在世界坐标系下的表示
    % alpha_deg 是角度阈值，单位为度
    % current_mode 是无人机当前的模式，'N' 或 'S'
    
    % 计算当前夹角的余弦值
    cos_theta = -c;  % 因为世界坐标系z轴是(0, 0, -1)

    % 将角度阈值从度转换为余弦值
    cos_alpha = cosd(alpha_deg);

    % 根据当前模式和夹角的余弦值决定是否切换模式
    if current_mode == 'N' && cos_theta < cos_alpha
        % 如果当前是N模式且夹角小于阈值，切换到S模式
        mode = 'S';
    elseif current_mode == 'S' && cos_theta > -cos_alpha
        % 如果当前是S模式且夹角大于阈值，切换到N模式
        mode = 'N';
    else
        % 否则保持当前模式不变
        mode = current_mode;
    end
end

== matlab function summary/MATLAB Function1 ==
  data: f input; w1 output; tau_x input; tau_y input; w2 output; w3 output; tau_z input; w4 output; C_T input; C_M input; p input; D_p input; D input; Eta input
function [w1, w2, w3, w4] = converter(f, tau_x, tau_y, tau_z, C_T, C_M, p, D_p, D, Eta)
% Convert thrust and torque to motor speeds
% Required parameters: thrust coefficient C_T, torque coefficient C_M, air density ρ, propeller diameter D_p,
% UAV arm length D, maximum thrust f_max, maximum torque tau_max

% f = min(f, f_max);
% tau_x = min(tau_x, tau_max);
% tau_y = min(tau_y, tau_max);
% tau_z = min(tau_z, tau_max);

a = [f; tau_x; tau_y; tau_z];

A = [C_T*p*D_p^4/(4*pi^2), C_T*p*D_p^4/(4*pi^2), C_T*p*D_p^4/(4*pi^2), C_T*p*D_p^4/(4*pi^2); 
    sqrt(2)/2*D*C_T*p*D_p^4/(4*pi^2), -sqrt(2)/2*D*C_T*p*D_p^4/(4*pi^2), -sqrt(2)/2*D*C_T*p*D_p^4/(4*pi^2), sqrt(2)/2*D*C_T*p*D_p^4/(4*pi^2);
    sqrt(2)/2*D*C_T*p*D_p^4/(4*pi^2), sqrt(2)/2*D*C_T*p*D_p^4/(4*pi^2), -sqrt(2)/2*D*C_T*p*D_p^4/(4*pi^2), -sqrt(2)/2*D*C_T*p*D_p^4/(4*pi^2);
    C_M*p*D_p^5/(4*pi^2), -C_M*p*D_p^5/(4*pi^2), C_M*p*D_p^5/(4*pi^2), -C_M*p*D_p^5/(4*pi^2)];

b = A\a;

% 根据Eta处理转速
if Eta == 1
    % 计算实际的转速
    w1 = sqrt(abs(b(1)));
    w2 = sqrt(abs(b(2)));
    w3 = sqrt(abs(b(3)));
    w4 = sqrt(abs(b(4)));
elseif Eta == -1
    % 计算实际的转速
    w1 = -sqrt(abs(b(1)));
    w2 = -sqrt(abs(b(2)));
    w3 = -sqrt(abs(b(3)));
    w4 = -sqrt(abs(b(4)));
else
    % Default values if Eta is neither 1 nor -1
    w1 = 0;
    w2 = 0;
    w3 = 0;
    w4 = 0;
end

end
